simulink library "Springs_Axle1"  (R2026a)
settings: Solver=VariableStepAuto
undefined symbols (not defined in the file): Vehicle
libraries: sm_car_lib x1, Springs_Axle1_Independent x1, Springs_Axle1_Interconnected x1, Springs_Axle1_Linear x1, Springs_Axle1_None x1
Description:
  | Component of Simscape Vehicle Templates Library
  | 
  | Copyright 2018-2026 The MathWorks, Inc.
settings Model: Creator=smiller  LastModifiedBy=smiller

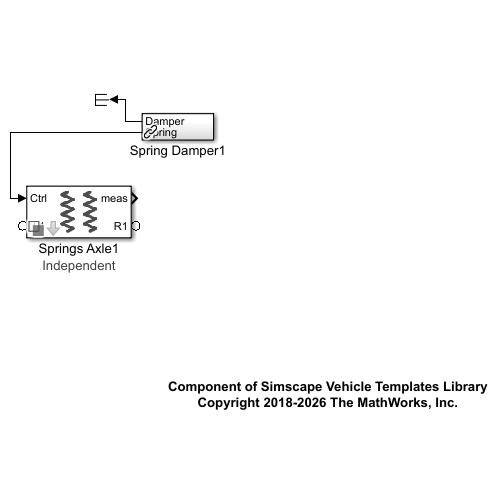
[thumbnail: Simulink's stored preview of the top-level diagram]
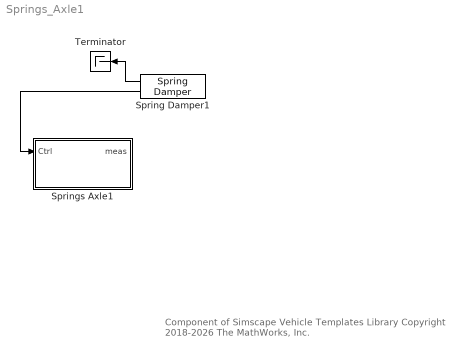
== system Springs_Axle1 ==
  note: Component of Simscape Vehicle Templates Library
      | Copyright 2018-2026 The MathWorks, Inc.
  Spring Damper1 : sm_car_lib/Inputs/Control Bus/Spring Damper  SystemSampleTime=-1  VariantActivationTime=update diagram  EmptyChoice=off  PassThrough=off  PassThroughVariantControl=(default)  EmptyChoiceVariantControl=(default)  AllowFlexibleInterface=on  Latency=0  AutoFrameSizeCalculation=off
  Springs Axle1 : Subsystem  Variant=on  VariantControlMode=label  VariantControl=Variant1  LabelModeActiveChoice=Independent  mask(Variants for Springs){Spring=Vehicle.Chassis.Spring, VariantLabel=Vehicle.Chassis.Spring.class.Value, InitTriggerDropdown=1}
      mask prompts: Spring "Spring Parameters"; VariantLabel "Variant Label"; InitTriggerDropdown "Initialization Trigger Dropdown"
      mask help: Select option and provide parameters for left and right springs. Option is chosen by string provided in Variant Label. The parameters for the selected option is contained in Springs data structure.
      mask init:
      | curblk = gcb;
      | 
      | % Set variant for this block 
      | set_param(curblk,'LabelModeActiveChoice',VariantLabel);
      | 
      | % Trigger Mask Initialization for 
      | % variant subsystems below this level
      | sm_car_lib_maskInitTrigger(curblk);
      settings: AttributesFormatString=%<ActiveVariant>
      mask TypeOptions InitTriggerDropdown: 0 | 1
      mask Display:
      | if(strcmp(get_param(gcb,'LabelModeActiveChoice'),'None'))
      |     disp(' ');
      | else
      |     image('sm_car_vehicle_chassis_spring_IMAGE.png');
      | end
  Terminator : Terminator
  wires:
  Spring Damper1/1 -> Terminator/1
  Spring Damper1/2 -> Springs Axle1/1("Ctrl ")

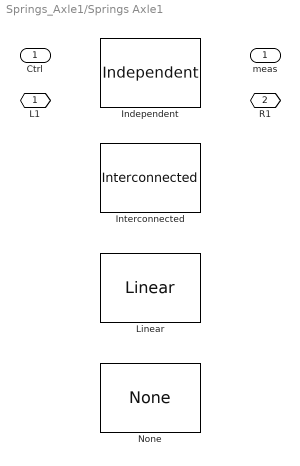
== system Springs_Axle1/Springs Axle1 ==
  "Ctrl " : Inport
  Independent : Springs_Axle1_Independent/Independent  VariantControl=Independent  InitTriggerDropdown=1
  Interconnected : Springs_Axle1_Interconnected/Interconnected  VariantControl=Interconnected  InitTriggerDropdown=1
  Linear : Springs_Axle1_Linear/Linear  SystemSampleTime=-1  VariantControl=Linear  VariantActivationTime=update diagram  EmptyChoice=off  PassThrough=off  PassThroughVariantControl=(default)  EmptyChoiceVariantControl=(default)  AllowFlexibleInterface=on  Latency=0  AutoFrameSizeCalculation=off
  None : Springs_Axle1_None/None  VariantControl=None  InitTriggerDropdown=1
  " L1" : PMIOPort  Side=Left
  R1 : PMIOPort  Port=2  Side=Right
  " meas" : Outport  VectorParamsAs1DForOutWhenUnconnected=off
